simulink model "Exe_L4_PartI"  (R2020a)
settings: Solver=VariableStepAuto  StartTime=0.0  StopTime=1  FixedStep=Ts  RelTol=1e-3  AbsTol=1e-3
InitFcn:
  | Ts=0.001;
  | %%
  | r1 = 8.05e-5;
  | r2 = -2.5e-7;
  | s = 0.185;
  | t1 = 1.002;
  | t2 = 8.424;
  | t3 = 247.3;
  | A = 0.25;%(m2)
  | Ct = 6000000/3600;%# Heat capacity of electrolyzer (Wh/K)
  | Ct1 = 46.7;%# Heat capacity of electrolyzer (Wh/K)
  | Rt = 0.018; % Heat resistance of electrolyzer(K/W)
  | Rt1 = 0.2; % Heat resistance of electrolyzer(K/W)
  | Ncell = 80; %   Number of cell each stack
  | Tmax = 273.15 + 80; % Max. stack temperature (K)
  | Ta = 20+273.15; % Ambient temperature (K)
  | Tini = 273.15 + 20; % Initial temperature(K)
libraries: powerlib x15, powerlib_meascontrol x8
Description:
  | Copyright 2008-2011 The MathWorks, Inc.
settings Model: FPTRunName=Active  ExtModeTrigMode=oneshot  ExtModeArmWhenConnect=off  ExtModeAutoUpdateStatusClock=off  Creator=MathWorks  LastModifiedBy=chunhua
settings SolverCC: AutoScaleAbsTol=off
settings DataIOCC: SaveFormat=Array  SaveOutput=off  SaveTime=off  ReturnWorkspaceOutputs=off  SignalLoggingName=sigsOut
settings OptimizationCC: BlockReduction=off  BooleanDataType=off  ExpressionDepthLimit=2147483647  InitFltsAndDblsToZero=on  EfficientMapNaN2IntZero=off  LifeSpan=inf
settings DebuggingCC: SaveWithParameterizedLinksMsg=none  UnderspecifiedInitializationDetection=Classic  MergeDetectMultiDrivingBlocksExec=none  CheckExecutionContextPreStartOutputMsg=on  CheckExecutionContextRuntimeOutputMsg=on  SignalResolutionControl=TryResolveAllWithWarning  MultiTaskDSMMsg=warning  MultiTaskCondExecSysMsg=none  FcnCallInpInsideContextMsg=warning  StateNameClashWarn=warning  SFUnexpectedBacktrackingDiag=warning  SFNoUnconditionalDefaultTransitionDiag=warning  SFExecutionAtInitializationDiag=none  ArithmeticOperatorsInVariantConditions=warning
settings HardwareCC: ProdBitPerPointer=32  ProdBitPerSizeT=32  ProdBitPerPtrDiffT=32  ProdLargestAtomicFloat=None  ProdIntDivRoundTo=Undefined  ProdEndianess=Unspecified  ProdWordSize=32  ProdHWDeviceType=32-bit Generic  TargetUnknown=on
settings ModelReferenceCC: PropagateSignalLabelsOutOfModel=off
settings SFSimCC: SimUseLocalCustomCode=off  CustomCodeUndefinedFunction=UseInterfaceOnly
settings RTWCC: RTWUseLocalCustomCode=off
settings CodeAppCC: StateflowObjectComments=on
settings GRTTargetCC: TargetFcnLib=ansi_tfl_tmw.mat  TargetLangStandard=C89/C90 (ANSI)  CombineOutputUpdateFcns=off  GRTInterface=on
settings ConfigComp: CovMetricSettings=dw  CovHtmlReporting=on  CovSaveCumulativeToWorkspaceVar=on  CovSaveSingleToWorkspaceVar=on  CovExternalEMLEnable=off
settings SimscapeCC: SimscapeNormalizeSystem=off

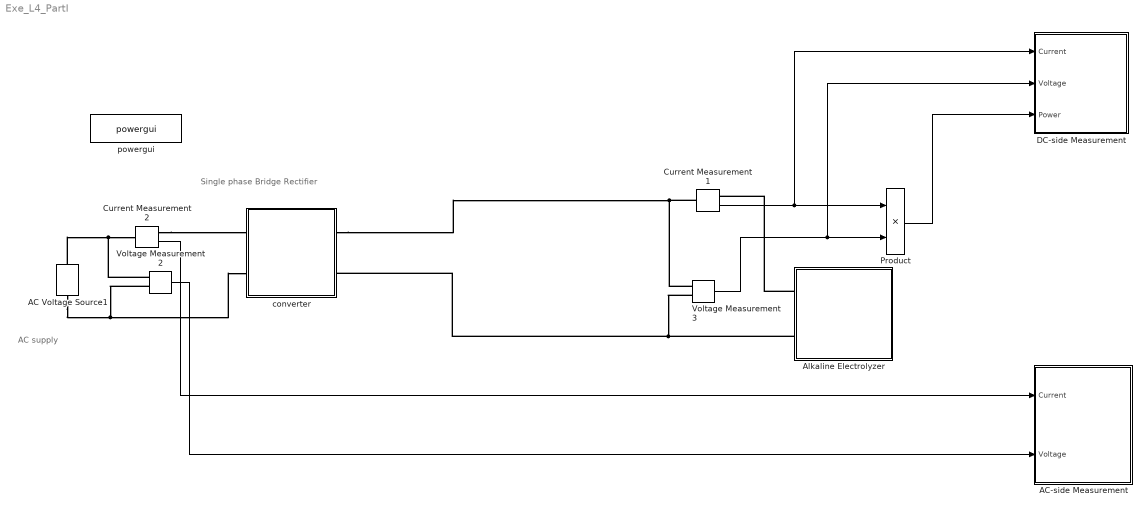
== system Exe_L4_PartI ==
  note: Single phase Bridge Rectifier
  note: AC supply
  AC Voltage Source1 : powerlib/Electrical Sources/AC Voltage Source  Amplitude=250  Phase=0  Frequency=50  SampleTime=5e-5  Measurements=None  BusType=swing  Pref=10e3  Qref=0  Qmin=-inf  Qmax=+inf
  AC-side Measurement : Subsystem
  Alkaline Electrolyzer : Subsystem
  Current Measurement1 : powerlib/Measurements/Current Measurement  PhasorSimulation=off  OutputType=Complex  PSBequivalent=0
  Current Measurement2 : powerlib/Measurements/Current Measurement  PhasorSimulation=off  OutputType=Complex  PSBequivalent=0
  DC-side Measurement : Subsystem
  Product : Product
  Voltage Measurement2 : powerlib/Measurements/Voltage Measurement  PhasorSimulation=off  OutputType=Complex  PSBequivalent=0
  Voltage Measurement3 : powerlib/Measurements/Voltage Measurement  PhasorSimulation=off  OutputType=Complex  PSBequivalent=0
  converter : Subsystem
  powergui : powerlib/powergui  Priority=1  SimulationMode=Discrete  SampleTime=1e-3  frequency=60  Iterations=50  frequencyindice=0  Pbase=100e6  ErrMax=1e-4  UnitsV=kV  UnitsW=MW  buscounter=0  FunctionMessages=off  echomessages=off  EnableUseOfTLC=off  CurrentSourceSwitches=off  DisableSnubberDevices=off  DisableRonSwitches=off  DisableVfSwitches=off  DisplayEquations=off  AutomaticDiscreteSolvers=off  SolverType=Tustin/Backward Euler (TBE)  Interpol=off  ExternalGateDelay=off  methode=off  Ts=0  x0status=blocks  SPID=off  SwTol=0  HookPort=off  NonlinearTolerance=1e-4  nMaxIteration=100  ContinueOnMaxIteration=off  RestoreLinks=warning  ResistiveCurrentMeasurement=off  Frange=[0:2:500]  Ylog=off  Xlog=on  ShowGrid=off  save=off  variable=ZData  structure=SPBR_R  ZoomFFT=off  StartTime=0.0  cycles=1  DisplayStyle=1  fundamental=100  FreqAxis=off  MaxFrequency=1000  frequencyindicesteady=1  RmsSteady=1  display=off
  wires:
  Product/1 -> DC-side Measurement/3(Power)
  Voltage Measurement2/1 -> AC-side Measurement/2(Voltage)
  Voltage Measurement3/1 -> DC-side Measurement/2(Voltage), Product/2
  Current Measurement1/1 -> DC-side Measurement/1(Current), Product/1
  Current Measurement2/1 -> AC-side Measurement/1(Current)
  connections:
  Alkaline Electrolyzer/LConn1 -- Current Measurement1/RConn1
  Voltage Measurement3/LConn1 -- converter/RConn1 -- Current Measurement1/LConn1
  converter/RConn2 -- Voltage Measurement3/LConn2 -- Alkaline Electrolyzer/LConn2
  Current Measurement2/RConn1 -- converter/LConn1
  AC Voltage Source1/RConn1 -- Voltage Measurement2/LConn1 -- Current Measurement2/LConn1
  AC Voltage Source1/LConn1 -- Voltage Measurement2/LConn2 -- converter/LConn2

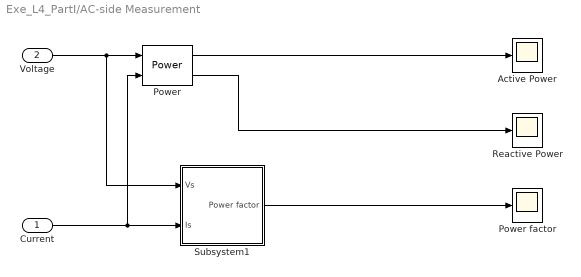
== system Exe_L4_PartI/AC-side Measurement ==
  Current : Inport
  Voltage : Inport  Port=2
  Active Power : Scope
  Power : powerlib_meascontrol/Measurements/Power  Freq=50  Vinit=[1, 0]  Iinit=[1, 0]  Ts=0
  Power factor : Scope
  Reactive Power : Scope
  Subsystem1 : Subsystem
  wires:
  Voltage/1 -> Subsystem1/1(Vs), Power/1
  Power/2 -> Reactive Power/1
  Current/1 -> Power/2, Subsystem1/2(Is)
  Power/1 -> Active Power/1
  Subsystem1/1(Power factor) -> Power factor/1

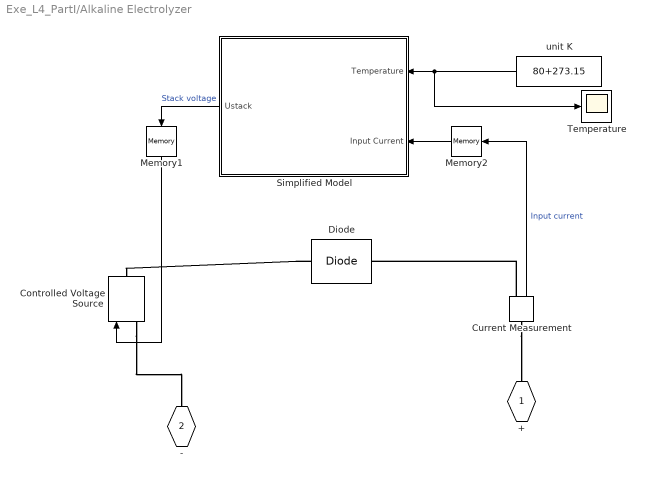
== system Exe_L4_PartI/Alkaline Electrolyzer ==
  Controlled Voltage Source : powerlib/Electrical Sources/Controlled Voltage Source  Initialize=on  Source_Type=DC  Amplitude=0  Phase=0  Frequency=0  Measurements=None
  Current Measurement : powerlib/Measurements/Current Measurement  PhasorSimulation=off  OutputType=Complex  PSBequivalent=0
  Diode : powerlib/Power Electronics/Diode  Ron=0.001  Lon=0  Vf=0.001  IC=0  UseSnubber=0  Rs=1000  Cs=0  Measurements=off
  Memory1 : Memory  InitialCondition=6
  Memory2 : Memory  InitialCondition=6
  Simplified Model : Subsystem
      settings: PortSchema="{\"entries\":[{\"content\":{\"sides\":[{\"content\":{\"connectorIds\":[\"Out1\"]},\"type\":\"ConnectorPlacement.EquallySpacedRectSide\",\"uuid\":\"5f83ef6f-0589-482a-9b32-d20637e9aaa8\"},{\"content\":{\"connectorIds\":[\"In1\",\"In2\"],\"side\":\"RIGHT\"},\"type\":\"ConnectorPlacement.EquallySpacedRectSide\",\"uuid\":\"bd19202e-8fd7-4998-8624-3fadad929c5b\"},{\"content\":{\"connectorIds\":[],\"side\":\"TOP\"},\"type\":\"ConnectorPlacement.EquallySpacedRectSide\",\"uuid\":\"98f7d102-06ad-4233-ab6e-a74ae6e9b1b4\"}]},\"type\":\"ConnectorPlacement.EquallySpacedConnector\",\"uuid\":\"8bdd7876-b33b-4755-8462-9551e25ec59e\"}],\"packageUris\":[\"http://schema.mathworks.com/mf0/Connector/19700101\"],\"version\":\"1.0\"}"
  Temperature : Scope
  unit K : Constant  Value=80+273.15  SampleTime=-1
  + : PMIOPort  Tag=PMCPort  Side=Left
  - : PMIOPort  Tag=PMCPort  Port=2  Side=Left
  wires:
  Current Measurement/1 -> Memory2/1  "Input current"
  unit K/1 -> Temperature/1, Simplified Model/1(Temperature)
  Simplified Model/1(Ustack) -> Memory1/1  "Stack voltage"
  Memory1/1 -> Controlled Voltage Source/1
  Memory2/1 -> Simplified Model/2(Input Current)
  connections:
  Current Measurement/LConn1 -- +/RConn1
  Diode/RConn1 -- Controlled Voltage Source/RConn1
  Current Measurement/RConn1 -- Diode/LConn1
  Controlled Voltage Source/LConn1 -- -/RConn1

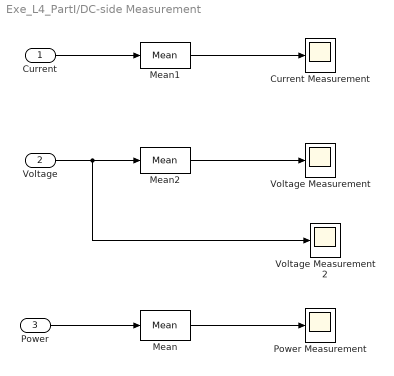
== system Exe_L4_PartI/DC-side Measurement ==
  Current : Inport
  Voltage : Inport  Port=2
  Power : Inport  Port=3
  Current Measurement : Scope
  Mean : powerlib_meascontrol/Measurements/Mean  Freq=50  Vinit=0  Ts=0
  Mean1 : powerlib_meascontrol/Measurements/Mean  Freq=50  Vinit=0  Ts=0
  Mean2 : powerlib_meascontrol/Measurements/Mean  Freq=50  Vinit=0  Ts=0
  Power Measurement : Scope
  Voltage Measurement : Scope
  Voltage Measurement 2 : Scope
  wires:
  Mean2/1 -> Voltage Measurement/1
  Mean1/1 -> Current Measurement/1
  Current/1 -> Mean1/1
  Voltage/1 -> Voltage Measurement 2/1, Mean2/1
  Power/1 -> Mean/1
  Mean/1 -> Power Measurement/1

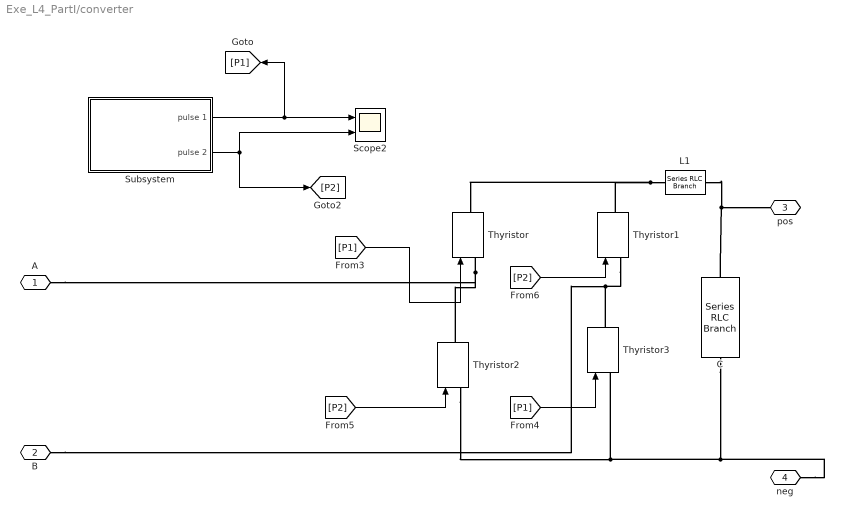
== system Exe_L4_PartI/converter ==
  C : powerlib/Elements/Series RLC Branch  LConnTagsString=__new0  RConnTagsString=__new0  BranchType=C  Resistance=1  Inductance=1e-3  SetiL0=off  InitialCurrent=0  Capacitance=0.1e-6  Setx0=on  InitialVoltage=0  Measurements=None
  L1 : powerlib/Elements/Series RLC Branch  LConnTagsString=__new0  RConnTagsString=__new0  BranchType=RL  Resistance=0.1  Inductance=5e-3  SetiL0=off  InitialCurrent=0  Capacitance=1e-6  Setx0=off  InitialVoltage=0  Measurements=None
  Scope2 : Scope  NumInputPorts=2
  Subsystem : Subsystem  mask{f=50, Amp=1, alpha=0}
      mask prompts: f "Frequency"; Amp "Amplitude"; alpha "Alpha (degree)"
      mask Display:
      | fprintf('Single phase\nPulse Generator')
      | port_label('output',1,'P1')
      | port_label('output',2,'P2')
  Thyristor{,1..3} (4 alike) : powerlib/Power Electronics/Thyristor  Ron=0.001  Lon=0  Vf=0.8  IC=0  Rs=500  Cs=250e-9  Measurements=off
  A : PMIOPort  Side=Left
  B : PMIOPort  Port=2  Side=Left
  pos : PMIOPort  Port=3  Side=Right
  neg : PMIOPort  Port=4  Side=Right
  wires:
  [P2] -> Thyristor1/1
  [P1] -> Thyristor/1
  [P1] -> Thyristor3/1
  [P2] -> Thyristor2/1
  Subsystem/2(pulse 2) -> Scope2/2, [P2]
  Subsystem/1(pulse 1) -> [P1], Scope2/1
  connections:
  C/RConn1 -- neg/RConn1 -- Thyristor3/LConn1 -- Thyristor2/LConn1
  Thyristor/LConn1 -- Thyristor2/RConn1 -- A/RConn1
  L1/LConn1 -- Thyristor1/RConn1 -- Thyristor/RConn1
  L1/RConn1 -- pos/RConn1 -- C/LConn1
  Thyristor1/LConn1 -- B/RConn1 -- Thyristor3/RConn1

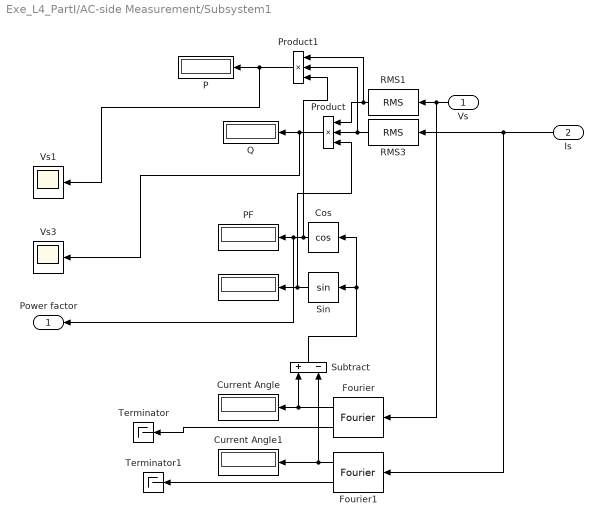
== system Exe_L4_PartI/AC-side Measurement/Subsystem1 ==
  Vs : Inport
  Is : Inport  Port=2
  "  " : Display
  Cos : Trigonometry  Operator=cos
  Current Angle : Display
  Current Angle1 : Display
  Fourier : powerlib_meascontrol/Measurements/Fourier  Freq=50  n=1  InInit=[0, 0]  Ts=5e-5
  Fourier1 : powerlib_meascontrol/Measurements/Fourier  Freq=50  n=1  InInit=[0, 0]  Ts=5e-5
  P : Display
  PF : Display
  Product : Product  Inputs=3
  Product1 : Product  Inputs=3
  Q : Display
  RMS1 : powerlib_meascontrol/Measurements/RMS  TrueRMS=on  Freq=50  RMSInit=120  Ts=0
  RMS3 : powerlib_meascontrol/Measurements/RMS  TrueRMS=on  Freq=50  RMSInit=120  Ts=0
  Sin : Trigonometry
  Subtract : Sum  Inputs=+-
  Terminator : Terminator
  Terminator1 : Terminator
  Vs1 : Scope
  Vs3 : Scope
  Power factor : Outport
  wires:
  Subtract/1 -> Sin/1, Cos/1
  Sin/1 -> Product/3, "  "/1
  RMS3/1 -> Product1/2, Product/2
  Cos/1 -> Product1/3, Power factor/1, PF/1
  Fourier/2 -> Current Angle/1, Subtract/1
  Product/1 -> Vs3/1, Q/1
  Fourier1/2 -> Current Angle1/1, Subtract/2
  RMS1/1 -> Product1/1, Product/1
  Fourier/1 -> Terminator/1
  Is/1 -> Fourier1/1, RMS3/1
  Vs/1 -> Fourier/1, RMS1/1
  Fourier1/1 -> Terminator1/1
  Product1/1 -> Vs1/1, P/1

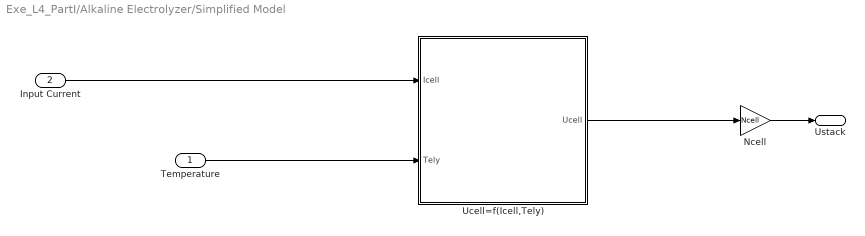
== system Exe_L4_PartI/Alkaline Electrolyzer/Simplified Model ==
  Temperature : Inport
  Input Current : Inport  Port=2
  Ncell : Gain  Gain=Ncell
  Ucell=f(Icell,Tely) : Subsystem
  Ustack : Outport  VectorParamsAs1DForOutWhenUnconnected=off
  wires:
  Input Current/1 -> Ucell=f(Icell,Tely)/1(Icell)
  Ucell=f(Icell,Tely)/1(Ucell) -> Ncell/1
  Ncell/1 -> Ustack/1
  Temperature/1 -> Ucell=f(Icell,Tely)/2(Tely)

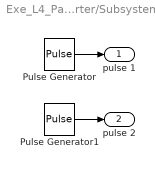
== system Exe_L4_PartI/converter/Subsystem ==
  Pulse Generator : DiscretePulseGenerator  PulseType=Time based  Amplitude=Amp  Period=1/f  PulseWidth=50  PhaseDelay=((1/f)/360)*alpha
  Pulse Generator1 : DiscretePulseGenerator  PulseType=Time based  Amplitude=Amp  Period=1/f  PulseWidth=50  PhaseDelay=(((1/f)/360)*alpha)+((1/f)/2)
  pulse 1 : Outport
  pulse 2 : Outport  Port=2
  wires:
  Pulse Generator/1 -> pulse 1/1
  Pulse Generator1/1 -> pulse 2/1

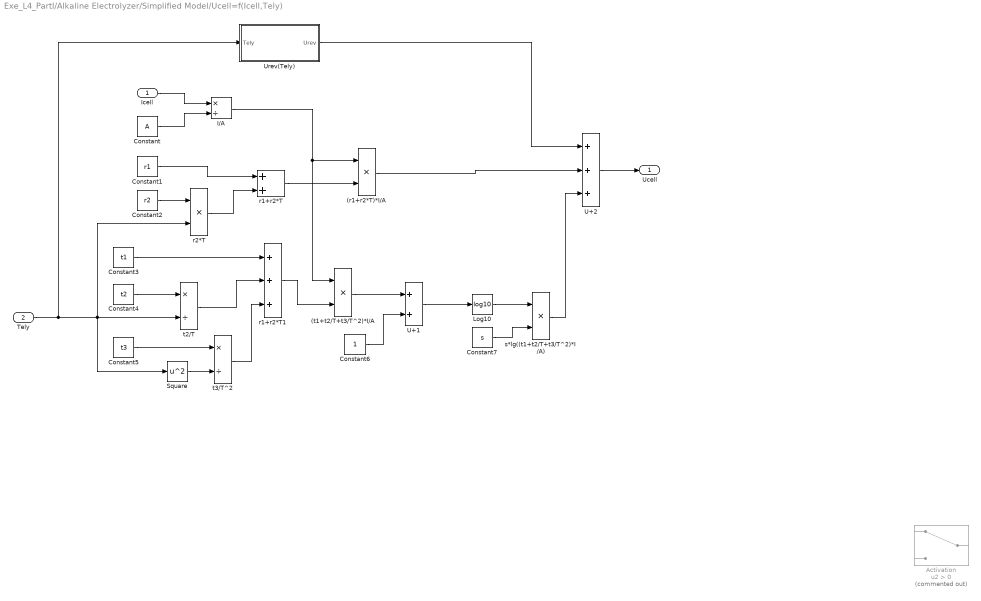
== system Exe_L4_PartI/Alkaline Electrolyzer/Simplified Model/Ucell=f(Icell,Tely) ==
  Icell : Inport
  Tely : Inport  Port=2
  (r1+r2*T)*I/A : Product
  (t1+t2/T+t3/T^2)*I/A : Product
  Activation : Switch  Commented=on  Criteria=u2 > Threshold
  Constant : Constant  Value=A
  Constant1 : Constant  Value=r1
  Constant2 : Constant  Value=r2
  Constant3 : Constant  Value=t1
  Constant4 : Constant  Value=t2
  Constant5 : Constant  Value=t3
  Constant6 : Constant
  Constant7 : Constant  Value=s
  I/A : Product  Inputs=*/
  Log10 : Math  Operator=log10  SignedPower=on  SaturateOnIntegerOverflow=on
  Square : Math  Operator=square  SignedPower=on  SaturateOnIntegerOverflow=on
  U+1 : Sum
  U+2 : Sum  Inputs=+++
  Urev(Tely) : MATLAB Function  TreatAsAtomicUnit=on
  r1+r2*T : Sum
  r1+r2*T1 : Sum  Inputs=+++
  r2*T : Product
  s*lg((t1+t2/T+t3/T^2)*I/A) : Product
  t2/T : Product  Inputs=*/
  t3/T^2 : Product  Inputs=*/
  Ucell : Outport
  wires:
  Constant5/1 -> t3/T^2/1
  Tely/1 -> Urev(Tely)/1(Tely), r2*T/2, t2/T/2, Square/1
  t2/T/1 -> r1+r2*T1/2
  r2*T/1 -> r1+r2*T/2
  Log10/1 -> s*lg((t1+t2/T+t3/T^2)*I/A)/1
  Constant/1 -> I/A/2
  Constant6/1 -> U+1/2
  (t1+t2/T+t3/T^2)*I/A/1 -> U+1/1
  Constant1/1 -> r1+r2*T/1
  I/A/1 -> (t1+t2/T+t3/T^2)*I/A/1, (r1+r2*T)*I/A/1
  Square/1 -> t3/T^2/2
  Constant4/1 -> t2/T/1
  Constant2/1 -> r2*T/1
  r1+r2*T/1 -> (r1+r2*T)*I/A/2
  Constant7/1 -> s*lg((t1+t2/T+t3/T^2)*I/A)/2
  Constant3/1 -> r1+r2*T1/1
  t3/T^2/1 -> r1+r2*T1/3
  r1+r2*T1/1 -> (t1+t2/T+t3/T^2)*I/A/2
  Icell/1 -> I/A/1
  U+2/1 -> Ucell/1
  (r1+r2*T)*I/A/1 -> U+2/2
  s*lg((t1+t2/T+t3/T^2)*I/A)/1 -> U+2/3
  U+1/1 -> Log10/1
  Urev(Tely)/1(Urev) -> U+2/1

== matlab function Exe_L4_PartI/Alkaline Electrolyzer/Simplified Model/Ucell=f(Icell,Tely)/Urev(Tely) ==
  data: Tely input; Urev output
function Urev = fcn(Tely)
Urev_t = 1.5184 - 1.5421e-3*Tely + 9.256e-5*Tely*log(Tely) + 9.84e-8*Tely^2;

Urev = Urev_t;
